simulink model "TCS_Simulation"  (R2023b)
settings: Solver=FixedStepAuto  StartTime=0.0  StopTime=5  FixedStep=0.03  RelTol=1e-3
undefined symbols (not defined in the file): Ion, Lithium, sigbuilder_block
libraries: spsMosfetLib x24, fl_lib x20, nesl_utility x19, sdl_lib x12, slpidlib x5, spsBatteryLib x4, spsSeriesRLCBranchLib x4, spsPermanentMagnetSynchronousMachineLib x4, spspowerguiLib x1
(part 1 of 3)
settings Model: Creator=hp  LastModifiedBy=ADMIN
settings DebuggingCC: UnconnectedInputMsg=warning  UnconnectedOutputMsg=warning  UnconnectedLineMsg=warning
settings ModelReferenceCC: EnableRefExpFcnMdlSchedulingChecks=on
settings RTWCC: DLArmComputeVersion=19.05

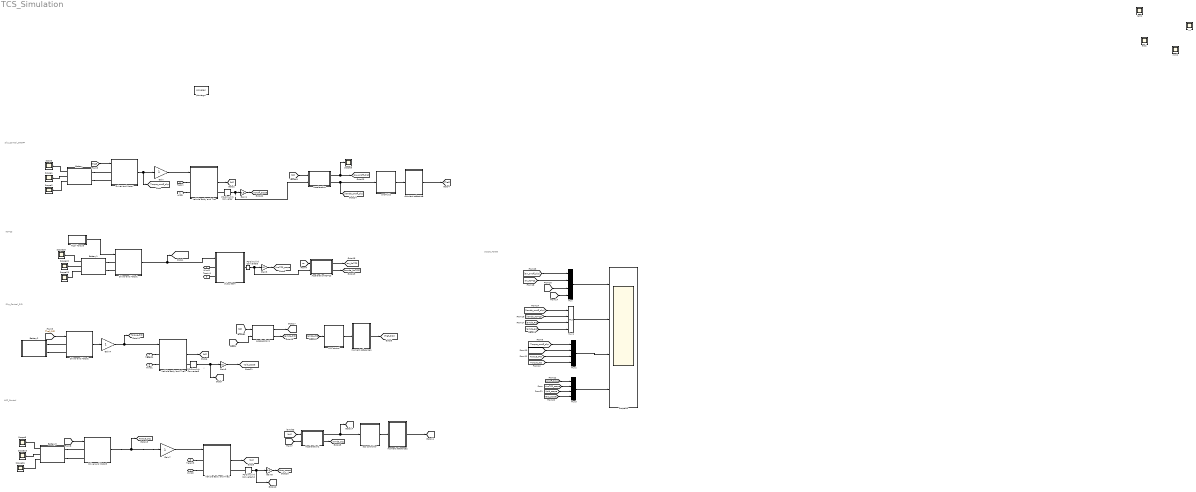
== system TCS_Simulation ==
  note: Scope_4Data
  note: Slip_Control_ONOFF
  note: NoTCS
  note: Slip_Control_PID
  note: ACC_Control
  note: v
  note: v
  Acceleration : Subsystem
  Acceleration1 : Subsystem
  Acceleration2 : Subsystem
  AccelerationNOTCS : Subsystem
  Battery : Subsystem
  Battery1 : Subsystem
  Battery2 : Subsystem
  Battery3 : Subsystem
  Driver and Motor : Subsystem
  Driver and Motor1 : Subsystem
  Driver and Motor2 : Subsystem
  Driver and Motor3 : Subsystem
  Gain : Gain
  Gain{1,3,5,8} (4 alike) : Gain  Gain=3.6
  Gain4 : Gain
  Gain7 : Gain
  High Torque : Subsystem  Tag=STV Subsys  LoadFcn=sigbuilder_block('load');  StartFcn=sigbuilder_block('start');  StopFcn=sigbuilder_block('stop');  ClipboardFcn=sigbuilder_block('clipboard');  mask(Sigbuilder block){tuvar=[0:10]}
      mask help: Simulink:masks:SigbuilderBlock_MD
      mask init:
      | if ~strcmp(get_param(bdroot(gcbh),'SimulationStatus'),'stopped') tuvar = sigbuilder_block('maskInit'); end
      settings: CopyFcn=sigbuilder_block('copy');  DeleteFcn=sigbuilder_block('delete');  ModelCloseFcn=sigbuilder_block('modelClose');  PreSaveFcn=sigbuilder_block('preSave');  PauseFcn=sigbuilder_block('pause');  ContinueFcn=sigbuilder_block('continue');  NameChangeFcn=sigbuilder_block('namechange');  OpenFcn=sigbuilder_block('open',[5.4 36 1141.2 516.6 ]);  CloseFcn=sigbuilder_block('close');
      mask Display: plot(0, 0, 100, 100,[2, 2, 32, 32, 2], [68, 8, 8, 68, 68],[32, 2], [38, 38], [32, 19, 2],[53, 60, 44], [32, 17, 17, 2],[16, 16, 31, 31]);txt = getActiveGroup(gcbh);text(2, 100, txt,'verticalAlignment', 'top');
  Mux{,1..3} (4 alike) : Mux
  PID control : Subsystem
  PS-Simulink Converter : nesl_utility/PS-Simulink Converter  PhysicalDomain=network_engine_domain  SubClassName=ps_output  LeftPortType=input  RightPortType=output  PseudoPeriodic=off  Frequencies=[]  VectorFormat=1-D array  Unit=1  AffineConversion=off
  PS-Simulink Converter12 : nesl_utility/PS-Simulink Converter  PhysicalDomain=network_engine_domain  SubClassName=ps_output  LeftPortType=input  RightPortType=output  PseudoPeriodic=off  Frequencies=[]  VectorFormat=1-D array  Unit=1  AffineConversion=off
  PS-Simulink Converter3 : nesl_utility/PS-Simulink Converter  PhysicalDomain=network_engine_domain  SubClassName=ps_output  LeftPortType=input  RightPortType=output  PseudoPeriodic=off  Frequencies=[]  VectorFormat=1-D array  Unit=inherit  AffineConversion=off
  PS-Simulink Converter8 : nesl_utility/PS-Simulink Converter  PhysicalDomain=network_engine_domain  SubClassName=ps_output  LeftPortType=input  RightPortType=output  PseudoPeriodic=off  Frequencies=[]  VectorFormat=1-D array  Unit=1  AffineConversion=off
  Scope{,1..3,8,16,18,22..23,26} (10 alike) : Scope
  Scope36 : Scope  NumInputPorts=4
  Subsystem : Subsystem
  Vehicle Body and Tire : Subsystem
  Vehicle Body and Tire1 : Subsystem
  Vehicle Body and Tire2 : Subsystem
  acc controller : Subsystem
  acc1 : Scope  NumInputPorts=4
  lam1 : Scope  NumInputPorts=4
  mm2 : Scope  NumInputPorts=4
  moment reference : Subsystem
  moment reference1 : Subsystem
  moment reference2 : Subsystem
  onoff slip : Subsystem
  powergui : spspowerguiLib/powergui  Priority=1  SimulationMode=Discrete  SampleTime=0.03  frequency=60  Iterations=50  frequencyindice=0  Pbase=100e6  ErrMax=1e-4  UnitsV=kV  UnitsW=MW  buscounter=0  FunctionMessages=off  echomessages=off  EnableUseOfTLC=off  CurrentSourceSwitches=off  DisableSnubberDevices=off  DisableRonSwitches=off  DisableVfSwitches=off  DisplayEquations=off  AutomaticDiscreteSolvers=off  SolverType=Tustin/Backward Euler (TBE)  Interpol=off  ExternalGateDelay=off  methode=off  Ts=10  x0status=blocks  SPID=off  SwTol=0  HookPort=off  NonlinearTolerance=1e-4  nMaxIteration=100  ContinueOnMaxIteration=off  RestoreLinks=warning  ResistiveCurrentMeasurement=off  Frange=[0:2:500]  Ylog=off  Xlog=on  ShowGrid=off  save=off  variable=ZData  structure=0  ZoomFFT=off  StartTime=0.0  cycles=1  DisplayStyle=1  fundamental=60  FreqAxis=off  MaxFrequency=1000  frequencyindicesteady=1  RmsSteady=1  display=off
  vv : Scope  NumInputPorts=4
  " Wind" : PMIOPort  Side=Left
  Terain : PMIOPort  Port=2  Side=Right
  Terain1 : PMIOPort  Port=3  Side=Left
  Wind1 : PMIOPort  Port=4  Side=Left
  " Wind1" : PMIOPort  Port=5  Side=Left
  Terain2 : PMIOPort  Port=6  Side=Right
  " Wind2" : PMIOPort  Port=7  Side=Left
  Terain3 : PMIOPort  Port=8  Side=Right
  tag scope: Torque_PID=global, Torque_acc=global, Torque_onoff_slip=global, VnoTCS_scope=global, Vonoff_Scope=global, Vpid_scope=global, aw_NoTCS=global, aw_PID=global, aw_acc=global, lamda_acc=global
  wires:
  moment reference/1(Tref) -> [Tref]
  Driver and Motor1/1(Torque) -> [Torque_NoTCS], Subsystem/1(Torque)
  Battery1/2(current) -> Scope22/1
  Battery1/3(Voltage) -> Scope23/1
  Battery/2(current) -> Scope1/1
  Battery1/1(SOC) -> Scope18/1
  [ss] -> AccelerationNOTCS/1(lamda1)
  [s1] -> Acceleration/1(lamda1)
  PS-Simulink Converter3/1 -> AccelerationNOTCS/2(Vx), Gain3/1
  Battery/1(SOC) -> Scope/1
  Gain/1 -> Vehicle Body and Tire/1(Torque)
  [Tref] -> Driver and Motor/1(Tref)
  PS-Simulink Converter/1 -> Acceleration/2(Vx), Gain1/1
  Driver and Motor/1(Torque) -> [Torque_onoff_slip], Gain/1
  Gain1/1 -> [Vonoff_Scope]
  Battery/3(Voltage) -> Scope2/1
  onoff slip/1(s) -> moment reference/1(S)
  Acceleration/2(lamda) -> [lamda_onoff_slip], onoff slip/1(lamda)
  AccelerationNOTCS/1(aw) -> [aw_NoTCS]
  AccelerationNOTCS/2(lamdaNoTCS) -> [lamda_NoTCS]
  Acceleration/1(aw) -> Scope3/1, [aw_onoff_slip]
  High Torque/1(Signal 1) -> Driver and Motor1/1(Tref)
  Vehicle Body and Tire/2(S) -> [s1]
  Vehicle Body and Tire1/2(s) -> [s2]
  Gain5/1 -> [Vpid_scope]
  PS-Simulink Converter8/1 -> [Vxpid], Gain5/1
  moment reference1/1(Tref) -> [Tref_PID]
  [Vxpid] -> Acceleration1/2(Vx)
  [Tref_PID] -> Driver and Motor2/1(Tref)
  Gain4/1 -> [Torque_PID], Vehicle Body and Tire1/1(Torque)
  Driver and Motor2/1(Torque) -> Gain4/1
  Acceleration1/2(lamda) -> [lamda_PID]
  PID control/1(s) -> moment reference1/1(S)
  [s2] -> Acceleration1/1(lamda1)
  Acceleration1/1(aw) -> [aw_PID]
  moment reference2/1(Tref) -> [Trefacc]
  [Vxacc] -> Acceleration2/2(Vx)
  Acceleration2/1(aw) -> acc controller/1(aw), [aw_acc]
  Battery3/3(Voltage) -> Scope26/1
  Vehicle Body and Tire2/2(s4) -> [s4]
  Acceleration2/2(lamda) -> [lamda_acc]
  PS-Simulink Converter12/1 -> Gain8/1, [Vxacc]
  Gain7/1 -> Vehicle Body and Tire2/1(Torque)
  acc controller/1(s) -> moment reference2/1(S)
  [s4] -> Acceleration2/1(lamda1)
  Battery3/2(current) -> Scope16/1
  Gain8/1 -> [Vacc_scope]
  [Trefacc] -> Driver and Motor3/1(Tref)
  Battery3/1(SOC) -> Scope8/1
  Driver and Motor3/1(Torque) -> Gain7/1, [Torque_acc]
  Mux/1 -> Scope36/1
  Mux1/1 -> Scope36/2
  Mux2/1 -> Scope36/3
  Mux3/1 -> Scope36/4
  [VnoTCS_scope] -> Mux3/2
  [Torque_onoff_slip] -> Mux2/1
  Gain3/1 -> [VnoTCS_scope]
  [Torque_NoTCS] -> Mux2/2
  [Torque_PID] -> Mux2/3
  [Torque_acc] -> Mux2/4
  [lamda_acc] -> Mux1/4
  [aw_acc] -> Mux/4
  [aw_PID] -> Mux/3
  [lamda_PID] -> PID control/1(lamda)
  [lamda_PID] -> Mux1/3
  [aw_NoTCS] -> Mux/2
  [lamda_NoTCS] -> Mux1/2
  [Vacc_scope] -> Mux3/4
  [Vpid_scope] -> Mux3/3
  [Vonoff_Scope] -> Mux3/1
  [aw_onoff_slip] -> Mux/1
  [lamda_onoff_slip] -> Mux1/1
  connections:
  Battery/LConn2 -- Driver and Motor/LConn2
  Battery/LConn1 -- Driver and Motor/LConn1
  " Wind"/RConn1 -- Vehicle Body and Tire/LConn2
  Terain/RConn1 -- Vehicle Body and Tire/LConn1
  PS-Simulink Converter/LConn1 -- Vehicle Body and Tire/RConn1
  Battery1/LConn1 -- Driver and Motor1/LConn1
  Battery1/LConn2 -- Driver and Motor1/LConn2
  Battery2/LConn2 -- Driver and Motor2/LConn2
  " Wind1"/RConn1 -- Vehicle Body and Tire1/LConn2
  Terain2/RConn1 -- Vehicle Body and Tire1/LConn1
  PS-Simulink Converter8/LConn1 -- Vehicle Body and Tire1/RConn1
  Battery2/LConn1 -- Driver and Motor2/LConn1
  Battery3/LConn1 -- Driver and Motor3/LConn1
  PS-Simulink Converter12/LConn1 -- Vehicle Body and Tire2/RConn1
  Battery3/LConn2 -- Driver and Motor3/LConn2
  " Wind2"/RConn1 -- Vehicle Body and Tire2/LConn2
  Terain3/RConn1 -- Vehicle Body and Tire2/LConn1
  Subsystem/RConn1 -- PS-Simulink Converter3/LConn1
  Subsystem/LConn1 -- Wind1/RConn1
  Subsystem/LConn2 -- Terain1/RConn1

== system TCS_Simulation/Acceleration ==
  note: W
  lamda1 : Inport
  Vx : Inport  Port=2
  Add : Sum
  Add1 : Sum  Inputs=+-
  Constant : Constant
  Derivative1 : Derivative
  Divide : Product  Inputs=*/
  Gain : Gain  Gain=1/0.22
  Product : Product
  Saturation : Saturate  UpperLimit=1  LowerLimit=0
  Scope1 : Scope
  Scope2 : Scope
  r : Gain  Gain=0.22
  wheel speed1 : Scope
  aw : Outport
  lamda : Outport  Port=2
  wires:
  Gain/1 -> r/1, wheel speed1/1
  lamda1/1 -> Product/1
  Product/1 -> Add/1
  r/1 -> Derivative1/1
  Constant/1 -> Add1/1
  Divide/1 -> Add1/2
  Add/1 -> Divide/2, Scope2/1, Gain/1
  Add1/1 -> Scope1/1, Saturation/1
  Vx/1 -> Divide/1, Add/2, Product/2
  Saturation/1 -> lamda/1
  Derivative1/1 -> aw/1

== system TCS_Simulation/Acceleration1 ==
  note: W
  lamda1 : Inport
  Vx : Inport  Port=2
  Add : Sum
  Add1 : Sum  Inputs=+-
  Constant : Constant
  Derivative1 : Derivative
  Divide : Product  Inputs=*/
  Gain : Gain  Gain=1/0.22
  Product : Product
  Saturation : Saturate  UpperLimit=1  LowerLimit=0
  Scope1 : Scope
  Scope2 : Scope
  r : Gain  Gain=0.22
  wheel speed1 : Scope
  aw : Outport
  lamda : Outport  Port=2
  wires:
  Gain/1 -> r/1, wheel speed1/1
  lamda1/1 -> Product/1
  Product/1 -> Add/1
  r/1 -> Derivative1/1
  Constant/1 -> Add1/1
  Divide/1 -> Add1/2
  Add/1 -> Divide/2, Scope2/1, Gain/1
  Add1/1 -> Scope1/1, Saturation/1
  Vx/1 -> Divide/1, Add/2, Product/2
  Saturation/1 -> lamda/1
  Derivative1/1 -> aw/1

== system TCS_Simulation/Acceleration2 ==
  note: W
  lamda1 : Inport
  Vx : Inport  Port=2
  Add : Sum
  Add1 : Sum  Inputs=+-
  Constant : Constant
  Derivative1 : Derivative
  Divide : Product  Inputs=*/
  Gain : Gain  Gain=1/0.22
  Product : Product
  Saturation : Saturate  UpperLimit=1  LowerLimit=0
  Scope1 : Scope
  Scope2 : Scope
  r : Gain  Gain=0.22
  wheel speed1 : Scope
  aw : Outport
  lamda : Outport  Port=2
  wires:
  Gain/1 -> r/1, wheel speed1/1
  lamda1/1 -> Product/1
  Product/1 -> Add/1
  r/1 -> Derivative1/1
  Constant/1 -> Add1/1
  Divide/1 -> Add1/2
  Add/1 -> Divide/2, Scope2/1, Gain/1
  Add1/1 -> Scope1/1, Saturation/1
  Vx/1 -> Divide/1, Add/2, Product/2
  Saturation/1 -> lamda/1
  Derivative1/1 -> aw/1

== system TCS_Simulation/AccelerationNOTCS ==
  note: Wr
  lamda1 : Inport
  Vx : Inport  Port=2
  Add : Sum
  Add1 : Sum  Inputs=+-
  Constant : Constant
  Derivative : Derivative
  Divide : Product  Inputs=*/
  Product : Product
  Scope1 : Scope
  Scope2 : Scope
  aw : Outport
  lamdaNoTCS : Outport  Port=2
  wires:
  Derivative/1 -> aw/1
  lamda1/1 -> Product/1
  Product/1 -> Add/1
  Add/1 -> Derivative/1, Divide/2, Scope2/1
  Constant/1 -> Add1/1
  Divide/1 -> Add1/2
  Add1/1 -> lamdaNoTCS/1
  Vx/1 -> Scope1/1, Divide/1, Product/2, Add/2

== system TCS_Simulation/Battery ==
  Battery : spsBatteryLib/Battery  BatType=Lithium-Ion  ShowTempParam=off  ThermalPreset=no  ShowAgeParam=off  NomV=50.4  NomQ=22  SOC=100  Batt_Tr=30  PresetModel=on  MaxQ=22  MinV=37.8  FullV=58.665  Dis_rate=9.5652  R=0.022909  Normal_OP=19.8957  expZone="[54.4514      1.08087]"  current=[6.5 13 32.5]  Units=Time  Tci=20  NomT=25  T2=0  MaxQ2=2.208  FullV2=3.45  Normal_OP2=2.8  expZone2="[3.22        0.23]"  Rca=0.6  ti=1000  Dp=0  Neq0=0  Tsim=1e6  Ta1=25  Qeol=5.4*0.9  Reol=0.013333*1.2  Char_age=[2.3478, 3]  Dis_age=[2.3478, 10]  N1=1500  N2=10500  N3=1000  N4=1400  Ta2=45  N5=950
  Bus Selector : BusSelector  OutputSignals=SOC (%),Current (A),Voltage (V)
  Series RLC Branch : spsSeriesRLCBranchLib/Series RLC Branch  LConnTagsString=__new0  RConnTagsString=__new0  BranchType=C  Resistance=1  Inductance=1e-3  SetiL0=off  InitialCurrent=0  Capacitance=75e-3  Setx0=off  InitialVoltage=0  Measurements=None
  " Positive" : PMIOPort  Side=Left
  Negative : PMIOPort  Port=2  Side=Left
  SOC : Outport
  current : Outport  Port=2
  Voltage : Outport  Port=3
  wires:
  Battery/1 -> Bus Selector/1
  Bus Selector/1 -> SOC/1  "<SOC (%)>"
  Bus Selector/2 -> current/1  "<Current (A)>"
  Bus Selector/3 -> Voltage/1  "<Voltage (V)>"
  connections:
  " Positive"/RConn1 -- Battery/LConn1 -- Series RLC Branch/LConn1
  Negative/RConn1 -- Series RLC Branch/RConn1 -- Battery/LConn2

== system TCS_Simulation/Battery1 ==
  Battery : spsBatteryLib/Battery  BatType=Lithium-Ion  ShowTempParam=off  ThermalPreset=no  ShowAgeParam=off  NomV=50.4  NomQ=22  SOC=100  Batt_Tr=30  PresetModel=on  MaxQ=22  MinV=37.8  FullV=58.665  Dis_rate=9.5652  R=0.022909  Normal_OP=19.8957  expZone="[54.4514      1.08087]"  current=[6.5 13 32.5]  Units=Time  Tci=20  NomT=25  T2=0  MaxQ2=2.208  FullV2=3.45  Normal_OP2=2.8  expZone2="[3.22        0.23]"  Rca=0.6  ti=1000  Dp=0  Neq0=0  Tsim=1e6  Ta1=25  Qeol=5.4*0.9  Reol=0.013333*1.2  Char_age=[2.3478, 3]  Dis_age=[2.3478, 10]  N1=1500  N2=10500  N3=1000  N4=1400  Ta2=45  N5=950
  Bus Selector : BusSelector  OutputSignals=SOC (%),Current (A),Voltage (V)
  Series RLC Branch : spsSeriesRLCBranchLib/Series RLC Branch  LConnTagsString=__new0  RConnTagsString=__new0  BranchType=C  Resistance=1  Inductance=1e-3  SetiL0=off  InitialCurrent=0  Capacitance=75e-3  Setx0=off  InitialVoltage=0  Measurements=None
  " Positive" : PMIOPort  Side=Left
  Negative : PMIOPort  Port=2  Side=Left
  SOC : Outport
  current : Outport  Port=2
  Voltage : Outport  Port=3
  wires:
  Battery/1 -> Bus Selector/1
  Bus Selector/1 -> SOC/1  "<SOC (%)>"
  Bus Selector/2 -> current/1  "<Current (A)>"
  Bus Selector/3 -> Voltage/1  "<Voltage (V)>"
  connections:
  " Positive"/RConn1 -- Battery/LConn1 -- Series RLC Branch/LConn1
  Negative/RConn1 -- Series RLC Branch/RConn1 -- Battery/LConn2

== system TCS_Simulation/Battery2 ==
  Battery : spsBatteryLib/Battery  BatType=Lithium-Ion  ShowTempParam=off  ThermalPreset=no  ShowAgeParam=off  NomV=50.4  NomQ=22  SOC=100  Batt_Tr=30  PresetModel=on  MaxQ=22  MinV=37.8  FullV=58.665  Dis_rate=9.5652  R=0.022909  Normal_OP=19.8957  expZone="[54.4514      1.08087]"  current=[6.5 13 32.5]  Units=Time  Tci=20  NomT=25  T2=0  MaxQ2=2.208  FullV2=3.45  Normal_OP2=2.8  expZone2="[3.22        0.23]"  Rca=0.6  ti=1000  Dp=0  Neq0=0  Tsim=1e6  Ta1=25  Qeol=5.4*0.9  Reol=0.013333*1.2  Char_age=[2.3478, 3]  Dis_age=[2.3478, 10]  N1=1500  N2=10500  N3=1000  N4=1400  Ta2=45  N5=950
  Bus Selector : BusSelector  OutputSignals=SOC (%),Current (A),Voltage (V)
  Series RLC Branch : spsSeriesRLCBranchLib/Series RLC Branch  LConnTagsString=__new0  RConnTagsString=__new0  BranchType=C  Resistance=1  Inductance=1e-3  SetiL0=off  InitialCurrent=0  Capacitance=75e-3  Setx0=off  InitialVoltage=0  Measurements=None
  " Positive" : PMIOPort  Side=Left
  Negative : PMIOPort  Port=2  Side=Left
  SOC : Outport
  current : Outport  Port=2
  Voltage : Outport  Port=3
  wires:
  Battery/1 -> Bus Selector/1
  Bus Selector/1 -> SOC/1  "<SOC (%)>"
  Bus Selector/2 -> current/1  "<Current (A)>"
  Bus Selector/3 -> Voltage/1  "<Voltage (V)>"
  connections:
  " Positive"/RConn1 -- Battery/LConn1 -- Series RLC Branch/LConn1
  Negative/RConn1 -- Series RLC Branch/RConn1 -- Battery/LConn2

== system TCS_Simulation/Battery3 ==
  Battery : spsBatteryLib/Battery  BatType=Lithium-Ion  ShowTempParam=off  ThermalPreset=no  ShowAgeParam=off  NomV=50.4  NomQ=22  SOC=100  Batt_Tr=30  PresetModel=on  MaxQ=22  MinV=37.8  FullV=58.665  Dis_rate=9.5652  R=0.022909  Normal_OP=19.8957  expZone="[54.4514      1.08087]"  current=[6.5 13 32.5]  Units=Time  Tci=20  NomT=25  T2=0  MaxQ2=2.208  FullV2=3.45  Normal_OP2=2.8  expZone2="[3.22        0.23]"  Rca=0.6  ti=1000  Dp=0  Neq0=0  Tsim=1e6  Ta1=25  Qeol=5.4*0.9  Reol=0.013333*1.2  Char_age=[2.3478, 3]  Dis_age=[2.3478, 10]  N1=1500  N2=10500  N3=1000  N4=1400  Ta2=45  N5=950
  Bus Selector : BusSelector  OutputSignals=SOC (%),Current (A),Voltage (V)
  Series RLC Branch : spsSeriesRLCBranchLib/Series RLC Branch  LConnTagsString=__new0  RConnTagsString=__new0  BranchType=C  Resistance=1  Inductance=1e-3  SetiL0=off  InitialCurrent=0  Capacitance=75e-3  Setx0=off  InitialVoltage=0  Measurements=None
  " Positive" : PMIOPort  Side=Left
  Negative : PMIOPort  Port=2  Side=Left
  SOC : Outport
  current : Outport  Port=2
  Voltage : Outport  Port=3
  wires:
  Battery/1 -> Bus Selector/1
  Bus Selector/1 -> SOC/1  "<SOC (%)>"
  Bus Selector/2 -> current/1  "<Current (A)>"
  Bus Selector/3 -> Voltage/1  "<Voltage (V)>"
  connections:
  " Positive"/RConn1 -- Battery/LConn1 -- Series RLC Branch/LConn1
  Negative/RConn1 -- Series RLC Branch/RConn1 -- Battery/LConn2

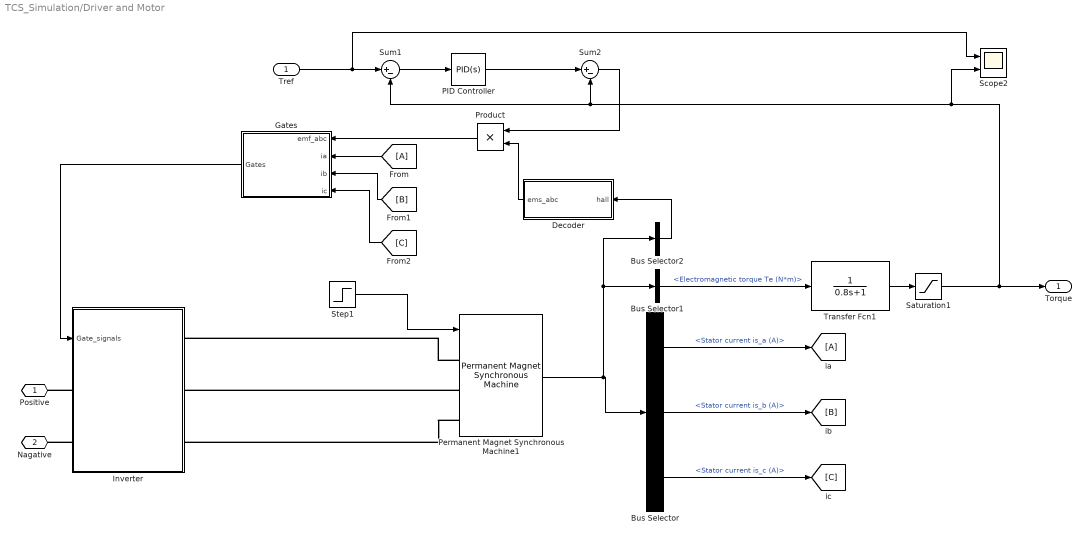
== system TCS_Simulation/Driver and Motor ==
  Tref : Inport
  Bus Selector : BusSelector  OutputSignals=Stator current is_a (A),Stator current is_b (A),Stator current is_c (A)
  Bus Selector1 : BusSelector  OutputSignals=Electromagnetic torque Te (N*m)
  Bus Selector2 : BusSelector  OutputSignals=Hall effect signal h_a,Hall effect signal h_b,Hall effect signal h_c  OutputAsBus=on
  Decoder : Subsystem
  From : From
  Gates : Subsystem
  Inverter : Subsystem
  PID Controller : slpidlib/PID Controller  Controller=PID  Form=Parallel  TimeDomain=Continuous-time  UseExternalTs=off  SampleTime=-1  IntegratorMethod=Forward Euler  FilterMethod=Forward Euler  ControllerParametersSource=internal  P=100  I=10  UseKiTs=off  D=1  N=100  UseFilter=on  TunerSelectOption=Transfer Function Based (PID Tuner App)  InitialConditionSource=internal  InitialConditionForIntegrator=0  InitialConditionForFilter=0  DifferentiatorICPrevScaledInput=0  ExternalReset=none  TrackingMode=off  Kt=1  LimitOutput=off  SatLimitsSource=internal  UpperSaturationLimit=inf  LowerSaturationLimit=-inf  LinearizeAsGain=on  AntiWindupMode=none  Kb=1  LimitIntegrator=off  UpperIntegratorSaturationLimit=inf  LowerIntegratorSaturationLimit=-inf  POutMin=[]  POutMax=[]  IOutMin=[]  IOutMax=[]  DOutMin=[]  DOutMax=[]  NOutMin=[]  NOutMax=[]  SumOutMin=[]  SumOutMax=[]  SaturationOutMin=[]  SaturationOutMax=[]  PParamMin=[]  PParamMax=[]  IParamMin=[]  IParamMax=[]  DParamMin=[]  DParamMax=[]  NParamMin=[]  NParamMax=[]  KbParamMin=[]  KbParamMax=[]  KtParamMin=[]  KtParamMax=[]  KbOutMin=[]  KbOutMax=[]  KtOutMin=[]  KtOutMax=[]  IntegratorOutMin=[]  IntegratorOutMax=[]  FilterOutMin=[]  FilterOutMax=[]  SumI1OutMin=[]  SumI1OutMax=[]  SumI2OutMin=[]  SumI2OutMax=[]  SumI3OutMin=[]  SumI3OutMax=[]  SumI4OutMin=[]  SumI4OutMax=[]  SumDOutMin=[]  SumDOutMax=[]  DifferentiatorOutMin=[]  DifferentiatorOutMax=[]  FilterDiffOutCoefMin=[]  FilterDiffOutCoefMax=[]  ReciprocalOutMin=[]  ReciprocalOutMax=[]  SumDenOutMin=[]  SumDenOutMax=[]  SumNumOutMin=[]  SumNumOutMax=[]  DivideOutMin=[]  DivideOutMax=[]  UdiffTsProdOutMin=[]  UdiffTsProdOutMax=[]  NTsProdOutMin=[]  NTsProdOutMax=[]  UintegralTsProdOutMin=[]  UintegralTsProdOutMax=[]  UngainTsProdOutMin=[]  UngainTsProdOutMax=[]  ClampingZeroOutDataTypeStr=Inherit: Inherit via back propagation  ClampingZeroOutMin=[]  ClampingZeroOutMax=[]  FilterDenConstantOutDataTypeStr=Inherit: Inherit via back propagation  FilterDenConstantOutMin=[]  FilterDenConstantOutMax=[]  PCopyOutDataTypeStr=Inherit: Inherit via back propagation  PCopyOutMin=[]  PCopyOutMax=[]  NCopyOutDataTypeStr=Inherit: Inherit via back propagation  NCopyOutMin=[]  NCopyOutMax=[]  IntegratorContinuousStateAttributes=''  IntegratorStateMustResolveToSignalObject=off  IntegratorRTWStateStorageClass=Auto  FilterContinuousStateAttributes=''  FilterStateMustResolveToSignalObject=off  FilterRTWStateStorageClass=Auto  ParallelPVariant=InternalParameters  IdealPVariant=Disabled  IVariant=InternalParameters  DVariant=InternalParameters  IntegratorVariant=Continuous  SatVariant=Disabled  AWVariant=Passthrough  PCopyVariant=Disabled  TRVariant=Disabled  FdbkBlocksVariant=Forward  IdealPFdbkVariant=Disabled  SatFdbkVariant=Disabled  DerivativeFilterVariant=ContFilter  NVariant=InternalParameters  NCopyVariant=Disabled  FilterICVariant=InternalICsFilter  IntegratorICVariant=InternalICs  ExternalResetVariant=Disabled  TRSumVariant=Passthrough  SumFdbkVariant=Disabled  SumVariant=Sum_PID  TsampFilterVariant=InternalTs  TsampNgainVariant=Passthrough  TsampIntegralVariant=Disabled_SignalSpec  ExternalSaturationOutDataTypeStr=Inherit: Same as second input
  Permanent Magnet Synchronous Machine1 : spsPermanentMagnetSynchronousMachineLib/Permanent Magnet Synchronous Machine  NbPhases=3  FluxDistribution=Trapezoidal  RotorType=Round  MechanicalLoad=Speed w  PresetModel=No  ShowDetailedParameters=on  MeasurementBus=off  Resistance=0.0485  Inductance=8.5e-3  dqInductances=[8.5e-3,8.5e-3]  La=0.000395  MachineConstant=Flux linkage established by magnets (V.s)  Flux=0.1194  VoltageCst=150.0425  TorqueCst=1.4328  Flat=120  Mechanical=[0.0027 0.0004924 4 0]  PolePairs=6  InitialConditions=[0,0, 0,0]  InitialConditions5ph=[0 0 0 0 0 0]  RefAngle=90 degrees behind phase A axis (modified Park)  IterativeDiscreteModel=Trapezoidal non iterative  TsBlock=-1  TsPowergui=0
  Product : Product
  Saturation1 : Saturate  UpperLimit=10000  LowerLimit=0
  Scope2 : Scope  NumInputPorts=2
  Step1 : Step  Time=100  After=200  SampleTime=0
  Sum1 : Sum  Inputs=|+-
  Sum2 : Sum  Inputs=|+-
  Transfer Fcn1 : TransferFcn  Denominator=[0.8 1]
  ia : Goto
  Positive : PMIOPort  Side=Left
  Nagative : PMIOPort  Port=2  Side=Left
  Torque : Outport
  wires:
  Bus Selector/3 -> [C]  "<Stator current is_c (A)>"
  Bus Selector2/1 -> Decoder/1(hall)
  [B] -> Gates/3(ib)
  Gates/1(Gates) -> Inverter/1(Gate_signals)
  Permanent Magnet Synchronous Machine1/1 -> Bus Selector1/1, Bus Selector2/1, Bus Selector/1
  Bus Selector/1 -> ia/1  "<Stator current is_a (A)>"
  Bus Selector/2 -> [B]  "<Stator current is_b (A)>"
  [C] -> Gates/4(ic)
  From/1 -> Gates/2(ia)
  Bus Selector1/1 -> Transfer Fcn1/1  "<Electromagnetic torque Te (N*m)>"
  Step1/1 -> Permanent Magnet Synchronous Machine1/1
  Decoder/1(ems_abc) -> Product/2
  Product/1 -> Gates/1(emf_abc)
  Sum1/1 -> PID Controller/1
  Tref/1 -> Scope2/1, Sum1/1
  PID Controller/1 -> Sum2/1
  Sum2/1 -> Product/1
  Transfer Fcn1/1 -> Saturation1/1
  Saturation1/1 -> Torque/1, Sum1/2, Sum2/2, Scope2/2
  connections:
  Inverter/LConn1 -- Positive/RConn1
  Inverter/LConn2 -- Nagative/RConn1
  Permanent Magnet Synchronous Machine1/LConn1 -- Inverter/RConn1
  Permanent Magnet Synchronous Machine1/LConn2 -- Inverter/RConn2
  Permanent Magnet Synchronous Machine1/LConn3 -- Inverter/RConn3

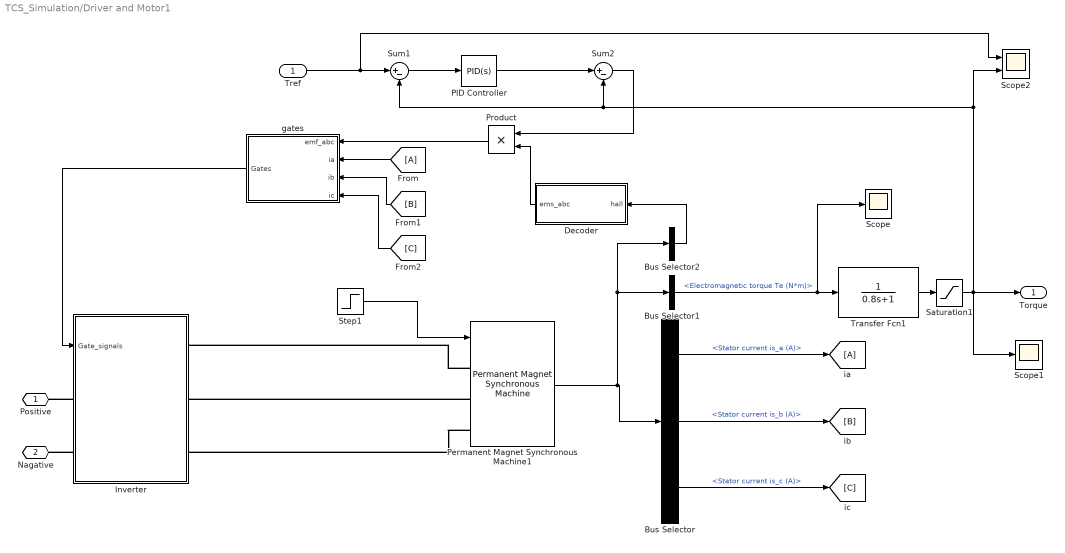
== system TCS_Simulation/Driver and Motor1 ==
  Tref : Inport
  Bus Selector : BusSelector  OutputSignals=Stator current is_a (A),Stator current is_b (A),Stator current is_c (A)
  Bus Selector1 : BusSelector  OutputSignals=Electromagnetic torque Te (N*m)
  Bus Selector2 : BusSelector  OutputSignals=Hall effect signal h_a,Hall effect signal h_b,Hall effect signal h_c  OutputAsBus=on
  Decoder : Subsystem
  From : From
  Inverter : Subsystem
  PID Controller : slpidlib/PID Controller  Controller=PID  Form=Parallel  TimeDomain=Continuous-time  UseExternalTs=off  SampleTime=-1  IntegratorMethod=Forward Euler  FilterMethod=Forward Euler  ControllerParametersSource=internal  P=100  I=10  UseKiTs=off  D=1  N=100  UseFilter=on  TunerSelectOption=Transfer Function Based (PID Tuner App)  InitialConditionSource=internal  InitialConditionForIntegrator=0  InitialConditionForFilter=0  DifferentiatorICPrevScaledInput=0  ExternalReset=none  TrackingMode=off  Kt=1  LimitOutput=off  SatLimitsSource=internal  UpperSaturationLimit=inf  LowerSaturationLimit=-inf  LinearizeAsGain=on  AntiWindupMode=none  Kb=1  LimitIntegrator=off  UpperIntegratorSaturationLimit=inf  LowerIntegratorSaturationLimit=-inf  POutMin=[]  POutMax=[]  IOutMin=[]  IOutMax=[]  DOutMin=[]  DOutMax=[]  NOutMin=[]  NOutMax=[]  SumOutMin=[]  SumOutMax=[]  SaturationOutMin=[]  SaturationOutMax=[]  PParamMin=[]  PParamMax=[]  IParamMin=[]  IParamMax=[]  DParamMin=[]  DParamMax=[]  NParamMin=[]  NParamMax=[]  KbParamMin=[]  KbParamMax=[]  KtParamMin=[]  KtParamMax=[]  KbOutMin=[]  KbOutMax=[]  KtOutMin=[]  KtOutMax=[]  IntegratorOutMin=[]  IntegratorOutMax=[]  FilterOutMin=[]  FilterOutMax=[]  SumI1OutMin=[]  SumI1OutMax=[]  SumI2OutMin=[]  SumI2OutMax=[]  SumI3OutMin=[]  SumI3OutMax=[]  SumI4OutMin=[]  SumI4OutMax=[]  SumDOutMin=[]  SumDOutMax=[]  DifferentiatorOutMin=[]  DifferentiatorOutMax=[]  FilterDiffOutCoefMin=[]  FilterDiffOutCoefMax=[]  ReciprocalOutMin=[]  ReciprocalOutMax=[]  SumDenOutMin=[]  SumDenOutMax=[]  SumNumOutMin=[]  SumNumOutMax=[]  DivideOutMin=[]  DivideOutMax=[]  UdiffTsProdOutMin=[]  UdiffTsProdOutMax=[]  NTsProdOutMin=[]  NTsProdOutMax=[]  UintegralTsProdOutMin=[]  UintegralTsProdOutMax=[]  UngainTsProdOutMin=[]  UngainTsProdOutMax=[]  ClampingZeroOutDataTypeStr=Inherit: Inherit via back propagation  ClampingZeroOutMin=[]  ClampingZeroOutMax=[]  FilterDenConstantOutDataTypeStr=Inherit: Inherit via back propagation  FilterDenConstantOutMin=[]  FilterDenConstantOutMax=[]  PCopyOutDataTypeStr=Inherit: Inherit via back propagation  PCopyOutMin=[]  PCopyOutMax=[]  NCopyOutDataTypeStr=Inherit: Inherit via back propagation  NCopyOutMin=[]  NCopyOutMax=[]  IntegratorContinuousStateAttributes=''  IntegratorStateMustResolveToSignalObject=off  IntegratorRTWStateStorageClass=Auto  FilterContinuousStateAttributes=''  FilterStateMustResolveToSignalObject=off  FilterRTWStateStorageClass=Auto  ParallelPVariant=InternalParameters  IdealPVariant=Disabled  IVariant=InternalParameters  DVariant=InternalParameters  IntegratorVariant=Continuous  SatVariant=Disabled  AWVariant=Passthrough  PCopyVariant=Disabled  TRVariant=Disabled  FdbkBlocksVariant=Forward  IdealPFdbkVariant=Disabled  SatFdbkVariant=Disabled  DerivativeFilterVariant=ContFilter  NVariant=InternalParameters  NCopyVariant=Disabled  FilterICVariant=InternalICsFilter  IntegratorICVariant=InternalICs  ExternalResetVariant=Disabled  TRSumVariant=Passthrough  SumFdbkVariant=Disabled  SumVariant=Sum_PID  TsampFilterVariant=InternalTs  TsampNgainVariant=Passthrough  TsampIntegralVariant=Disabled_SignalSpec  ExternalSaturationOutDataTypeStr=Inherit: Same as second input
  Permanent Magnet Synchronous Machine1 : spsPermanentMagnetSynchronousMachineLib/Permanent Magnet Synchronous Machine  NbPhases=3  FluxDistribution=Trapezoidal  RotorType=Round  MechanicalLoad=Speed w  PresetModel=No  ShowDetailedParameters=on  MeasurementBus=off  Resistance=0.0485  Inductance=8.5e-3  dqInductances=[8.5e-3,8.5e-3]  La=0.000395  MachineConstant=Flux linkage established by magnets (V.s)  Flux=0.1194  VoltageCst=150.0425  TorqueCst=1.4328  Flat=120  Mechanical=[0.0027 0.0004924 4 0]  PolePairs=6  InitialConditions=[0,0, 0,0]  InitialConditions5ph=[0 0 0 0 0 0]  RefAngle=90 degrees behind phase A axis (modified Park)  IterativeDiscreteModel=Trapezoidal non iterative  TsBlock=-1  TsPowergui=0
  Product : Product
  Saturation1 : Saturate  UpperLimit=10000  LowerLimit=0
  Scope : Scope
  Scope1 : Scope
  Scope2 : Scope  NumInputPorts=2
  Step1 : Step  Time=100  After=200  SampleTime=0
  Sum1 : Sum  Inputs=|+-
  Sum2 : Sum  Inputs=|+-
  Transfer Fcn1 : TransferFcn  Numerator=1  Denominator=[0.8 1]
  gates : Subsystem
  ia : Goto
  Positive : PMIOPort  Side=Left
  Nagative : PMIOPort  Port=2  Side=Left
  Torque : Outport
  wires:
  Bus Selector/3 -> [C]  "<Stator current is_c (A)>"
  Bus Selector2/1 -> Decoder/1(hall)
  [B] -> gates/3(ib)
  gates/1(Gates) -> Inverter/1(Gate_signals)
  Permanent Magnet Synchronous Machine1/1 -> Bus Selector1/1, Bus Selector2/1, Bus Selector/1
  Bus Selector/1 -> ia/1  "<Stator current is_a (A)>"
  Bus Selector/2 -> [B]  "<Stator current is_b (A)>"
  [C] -> gates/4(ic)
  From/1 -> gates/2(ia)
  Bus Selector1/1 -> Transfer Fcn1/1, Scope/1  "<Electromagnetic torque Te (N*m)>"
  Step1/1 -> Permanent Magnet Synchronous Machine1/1
  Decoder/1(ems_abc) -> Product/2
  Product/1 -> gates/1(emf_abc)
  Sum1/1 -> PID Controller/1
  Tref/1 -> Scope2/1, Sum1/1
  Transfer Fcn1/1 -> Saturation1/1
  PID Controller/1 -> Sum2/1
  Sum2/1 -> Product/1
  Saturation1/1 -> Torque/1, Sum1/2, Sum2/2, Scope2/2, Scope1/1
  connections:
  Inverter/LConn1 -- Positive/RConn1
  Inverter/LConn2 -- Nagative/RConn1
  Permanent Magnet Synchronous Machine1/LConn1 -- Inverter/RConn1
  Permanent Magnet Synchronous Machine1/LConn2 -- Inverter/RConn2
  Permanent Magnet Synchronous Machine1/LConn3 -- Inverter/RConn3

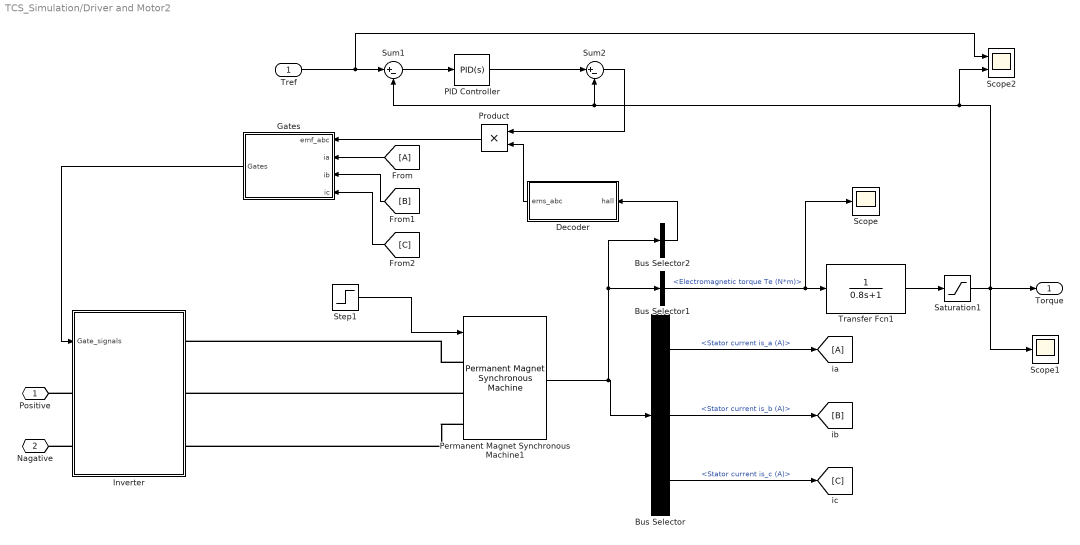
== system TCS_Simulation/Driver and Motor2 ==
  Tref : Inport
  Bus Selector : BusSelector  OutputSignals=Stator current is_a (A),Stator current is_b (A),Stator current is_c (A)
  Bus Selector1 : BusSelector  OutputSignals=Electromagnetic torque Te (N*m)
  Bus Selector2 : BusSelector  OutputSignals=Hall effect signal h_a,Hall effect signal h_b,Hall effect signal h_c  OutputAsBus=on
  Decoder : Subsystem
  From : From
  Gates : Subsystem
  Inverter : Subsystem
  PID Controller : slpidlib/PID Controller  Controller=PID  Form=Parallel  TimeDomain=Continuous-time  UseExternalTs=off  SampleTime=-1  IntegratorMethod=Forward Euler  FilterMethod=Forward Euler  ControllerParametersSource=internal  P=100  I=10  UseKiTs=off  D=1  N=100  UseFilter=on  TunerSelectOption=Transfer Function Based (PID Tuner App)  InitialConditionSource=internal  InitialConditionForIntegrator=0  InitialConditionForFilter=0  DifferentiatorICPrevScaledInput=0  ExternalReset=none  TrackingMode=off  Kt=1  LimitOutput=off  SatLimitsSource=internal  UpperSaturationLimit=inf  LowerSaturationLimit=-inf  LinearizeAsGain=on  AntiWindupMode=none  Kb=1  LimitIntegrator=off  UpperIntegratorSaturationLimit=inf  LowerIntegratorSaturationLimit=-inf  POutMin=[]  POutMax=[]  IOutMin=[]  IOutMax=[]  DOutMin=[]  DOutMax=[]  NOutMin=[]  NOutMax=[]  SumOutMin=[]  SumOutMax=[]  SaturationOutMin=[]  SaturationOutMax=[]  PParamMin=[]  PParamMax=[]  IParamMin=[]  IParamMax=[]  DParamMin=[]  DParamMax=[]  NParamMin=[]  NParamMax=[]  KbParamMin=[]  KbParamMax=[]  KtParamMin=[]  KtParamMax=[]  KbOutMin=[]  KbOutMax=[]  KtOutMin=[]  KtOutMax=[]  IntegratorOutMin=[]  IntegratorOutMax=[]  FilterOutMin=[]  FilterOutMax=[]  SumI1OutMin=[]  SumI1OutMax=[]  SumI2OutMin=[]  SumI2OutMax=[]  SumI3OutMin=[]  SumI3OutMax=[]  SumI4OutMin=[]  SumI4OutMax=[]  SumDOutMin=[]  SumDOutMax=[]  DifferentiatorOutMin=[]  DifferentiatorOutMax=[]  FilterDiffOutCoefMin=[]  FilterDiffOutCoefMax=[]  ReciprocalOutMin=[]  ReciprocalOutMax=[]  SumDenOutMin=[]  SumDenOutMax=[]  SumNumOutMin=[]  SumNumOutMax=[]  DivideOutMin=[]  DivideOutMax=[]  UdiffTsProdOutMin=[]  UdiffTsProdOutMax=[]  NTsProdOutMin=[]  NTsProdOutMax=[]  UintegralTsProdOutMin=[]  UintegralTsProdOutMax=[]  UngainTsProdOutMin=[]  UngainTsProdOutMax=[]  ClampingZeroOutDataTypeStr=Inherit: Inherit via back propagation  ClampingZeroOutMin=[]  ClampingZeroOutMax=[]  FilterDenConstantOutDataTypeStr=Inherit: Inherit via back propagation  FilterDenConstantOutMin=[]  FilterDenConstantOutMax=[]  PCopyOutDataTypeStr=Inherit: Inherit via back propagation  PCopyOutMin=[]  PCopyOutMax=[]  NCopyOutDataTypeStr=Inherit: Inherit via back propagation  NCopyOutMin=[]  NCopyOutMax=[]  IntegratorContinuousStateAttributes=''  IntegratorStateMustResolveToSignalObject=off  IntegratorRTWStateStorageClass=Auto  FilterContinuousStateAttributes=''  FilterStateMustResolveToSignalObject=off  FilterRTWStateStorageClass=Auto  ParallelPVariant=InternalParameters  IdealPVariant=Disabled  IVariant=InternalParameters  DVariant=InternalParameters  IntegratorVariant=Continuous  SatVariant=Disabled  AWVariant=Passthrough  PCopyVariant=Disabled  TRVariant=Disabled  FdbkBlocksVariant=Forward  IdealPFdbkVariant=Disabled  SatFdbkVariant=Disabled  DerivativeFilterVariant=ContFilter  NVariant=InternalParameters  NCopyVariant=Disabled  FilterICVariant=InternalICsFilter  IntegratorICVariant=InternalICs  ExternalResetVariant=Disabled  TRSumVariant=Passthrough  SumFdbkVariant=Disabled  SumVariant=Sum_PID  TsampFilterVariant=InternalTs  TsampNgainVariant=Passthrough  TsampIntegralVariant=Disabled_SignalSpec  ExternalSaturationOutDataTypeStr=Inherit: Same as second input
  Permanent Magnet Synchronous Machine1 : spsPermanentMagnetSynchronousMachineLib/Permanent Magnet Synchronous Machine  NbPhases=3  FluxDistribution=Trapezoidal  RotorType=Round  MechanicalLoad=Speed w  PresetModel=No  ShowDetailedParameters=on  MeasurementBus=off  Resistance=0.0485  Inductance=8.5e-3  dqInductances=[8.5e-3,8.5e-3]  La=0.000395  MachineConstant=Flux linkage established by magnets (V.s)  Flux=0.1194  VoltageCst=150.0425  TorqueCst=1.4328  Flat=120  Mechanical=[0.0027 0.0004924 4 0]  PolePairs=6  InitialConditions=[0,0, 0,0]  InitialConditions5ph=[0 0 0 0 0 0]  RefAngle=90 degrees behind phase A axis (modified Park)  IterativeDiscreteModel=Trapezoidal non iterative  TsBlock=-1  TsPowergui=0
  Product : Product
  Saturation1 : Saturate  UpperLimit=10000  LowerLimit=0
  Scope : Scope
  Scope1 : Scope
  Scope2 : Scope  NumInputPorts=2
  Step1 : Step  Time=100  After=200  SampleTime=0
  Sum1 : Sum  Inputs=|+-
  Sum2 : Sum  Inputs=|+-
  Transfer Fcn1 : TransferFcn  Denominator=[0.8 1]
  ia : Goto
  Positive : PMIOPort  Side=Left
  Nagative : PMIOPort  Port=2  Side=Left
  Torque : Outport
  wires:
  Bus Selector/3 -> [C]  "<Stator current is_c (A)>"
  Bus Selector2/1 -> Decoder/1(hall)
  [B] -> Gates/3(ib)
  Gates/1(Gates) -> Inverter/1(Gate_signals)
  Permanent Magnet Synchronous Machine1/1 -> Bus Selector1/1, Bus Selector2/1, Bus Selector/1
  Bus Selector/1 -> ia/1  "<Stator current is_a (A)>"
  Bus Selector/2 -> [B]  "<Stator current is_b (A)>"
  [C] -> Gates/4(ic)
  From/1 -> Gates/2(ia)
  Bus Selector1/1 -> Transfer Fcn1/1, Scope/1  "<Electromagnetic torque Te (N*m)>"
  Step1/1 -> Permanent Magnet Synchronous Machine1/1
  Decoder/1(ems_abc) -> Product/2
  Product/1 -> Gates/1(emf_abc)
  Sum1/1 -> PID Controller/1
  Tref/1 -> Scope2/1, Sum1/1
  PID Controller/1 -> Sum2/1
  Sum2/1 -> Product/1
  Transfer Fcn1/1 -> Saturation1/1
  Saturation1/1 -> Torque/1, Sum1/2, Sum2/2, Scope2/2, Scope1/1
  connections:
  Inverter/LConn1 -- Positive/RConn1
  Inverter/LConn2 -- Nagative/RConn1
  Permanent Magnet Synchronous Machine1/LConn1 -- Inverter/RConn1
  Permanent Magnet Synchronous Machine1/LConn2 -- Inverter/RConn2
  Permanent Magnet Synchronous Machine1/LConn3 -- Inverter/RConn3

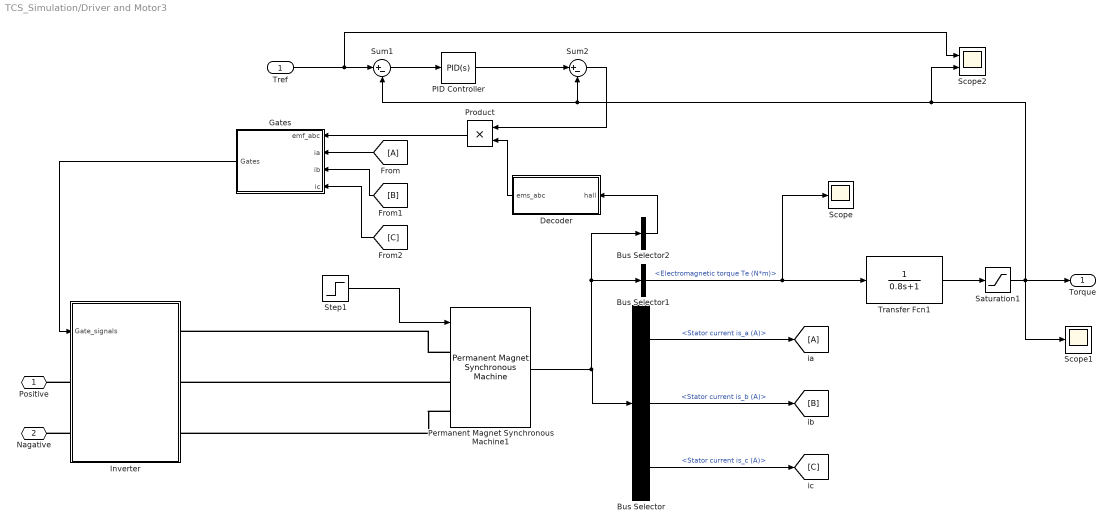
== system TCS_Simulation/Driver and Motor3 ==
  Tref : Inport
  Bus Selector : BusSelector  OutputSignals=Stator current is_a (A),Stator current is_b (A),Stator current is_c (A)
  Bus Selector1 : BusSelector  OutputSignals=Electromagnetic torque Te (N*m)
  Bus Selector2 : BusSelector  OutputSignals=Hall effect signal h_a,Hall effect signal h_b,Hall effect signal h_c  OutputAsBus=on
  Decoder : Subsystem
  From : From
  Gates : Subsystem
  Inverter : Subsystem
  PID Controller : slpidlib/PID Controller  Controller=PID  Form=Parallel  TimeDomain=Continuous-time  UseExternalTs=off  SampleTime=-1  IntegratorMethod=Forward Euler  FilterMethod=Forward Euler  ControllerParametersSource=internal  P=100  I=10  UseKiTs=off  D=1  N=100  UseFilter=on  TunerSelectOption=Transfer Function Based (PID Tuner App)  InitialConditionSource=internal  InitialConditionForIntegrator=0  InitialConditionForFilter=0  DifferentiatorICPrevScaledInput=0  ExternalReset=none  TrackingMode=off  Kt=1  LimitOutput=off  SatLimitsSource=internal  UpperSaturationLimit=inf  LowerSaturationLimit=-inf  LinearizeAsGain=on  AntiWindupMode=none  Kb=1  LimitIntegrator=off  UpperIntegratorSaturationLimit=inf  LowerIntegratorSaturationLimit=-inf  POutMin=[]  POutMax=[]  IOutMin=[]  IOutMax=[]  DOutMin=[]  DOutMax=[]  NOutMin=[]  NOutMax=[]  SumOutMin=[]  SumOutMax=[]  SaturationOutMin=[]  SaturationOutMax=[]  PParamMin=[]  PParamMax=[]  IParamMin=[]  IParamMax=[]  DParamMin=[]  DParamMax=[]  NParamMin=[]  NParamMax=[]  KbParamMin=[]  KbParamMax=[]  KtParamMin=[]  KtParamMax=[]  KbOutMin=[]  KbOutMax=[]  KtOutMin=[]  KtOutMax=[]  IntegratorOutMin=[]  IntegratorOutMax=[]  FilterOutMin=[]  FilterOutMax=[]  SumI1OutMin=[]  SumI1OutMax=[]  SumI2OutMin=[]  SumI2OutMax=[]  SumI3OutMin=[]  SumI3OutMax=[]  SumI4OutMin=[]  SumI4OutMax=[]  SumDOutMin=[]  SumDOutMax=[]  DifferentiatorOutMin=[]  DifferentiatorOutMax=[]  FilterDiffOutCoefMin=[]  FilterDiffOutCoefMax=[]  ReciprocalOutMin=[]  ReciprocalOutMax=[]  SumDenOutMin=[]  SumDenOutMax=[]  SumNumOutMin=[]  SumNumOutMax=[]  DivideOutMin=[]  DivideOutMax=[]  UdiffTsProdOutMin=[]  UdiffTsProdOutMax=[]  NTsProdOutMin=[]  NTsProdOutMax=[]  UintegralTsProdOutMin=[]  UintegralTsProdOutMax=[]  UngainTsProdOutMin=[]  UngainTsProdOutMax=[]  ClampingZeroOutDataTypeStr=Inherit: Inherit via back propagation  ClampingZeroOutMin=[]  ClampingZeroOutMax=[]  FilterDenConstantOutDataTypeStr=Inherit: Inherit via back propagation  FilterDenConstantOutMin=[]  FilterDenConstantOutMax=[]  PCopyOutDataTypeStr=Inherit: Inherit via back propagation  PCopyOutMin=[]  PCopyOutMax=[]  NCopyOutDataTypeStr=Inherit: Inherit via back propagation  NCopyOutMin=[]  NCopyOutMax=[]  IntegratorContinuousStateAttributes=''  IntegratorStateMustResolveToSignalObject=off  IntegratorRTWStateStorageClass=Auto  FilterContinuousStateAttributes=''  FilterStateMustResolveToSignalObject=off  FilterRTWStateStorageClass=Auto  ParallelPVariant=InternalParameters  IdealPVariant=Disabled  IVariant=InternalParameters  DVariant=InternalParameters  IntegratorVariant=Continuous  SatVariant=Disabled  AWVariant=Passthrough  PCopyVariant=Disabled  TRVariant=Disabled  FdbkBlocksVariant=Forward  IdealPFdbkVariant=Disabled  SatFdbkVariant=Disabled  DerivativeFilterVariant=ContFilter  NVariant=InternalParameters  NCopyVariant=Disabled  FilterICVariant=InternalICsFilter  IntegratorICVariant=InternalICs  ExternalResetVariant=Disabled  TRSumVariant=Passthrough  SumFdbkVariant=Disabled  SumVariant=Sum_PID  TsampFilterVariant=InternalTs  TsampNgainVariant=Passthrough  TsampIntegralVariant=Disabled_SignalSpec  ExternalSaturationOutDataTypeStr=Inherit: Same as second input
  Permanent Magnet Synchronous Machine1 : spsPermanentMagnetSynchronousMachineLib/Permanent Magnet Synchronous Machine  NbPhases=3  FluxDistribution=Trapezoidal  RotorType=Round  MechanicalLoad=Speed w  PresetModel=No  ShowDetailedParameters=on  MeasurementBus=off  Resistance=0.0485  Inductance=8.5e-3  dqInductances=[8.5e-3,8.5e-3]  La=0.000395  MachineConstant=Flux linkage established by magnets (V.s)  Flux=0.1194  VoltageCst=150.0425  TorqueCst=1.4328  Flat=120  Mechanical=[0.0027 0.0004924 4 0]  PolePairs=6  InitialConditions=[0,0, 0,0]  InitialConditions5ph=[0 0 0 0 0 0]  RefAngle=90 degrees behind phase A axis (modified Park)  IterativeDiscreteModel=Trapezoidal non iterative  TsBlock=-1  TsPowergui=0
  Product : Product
  Saturation1 : Saturate  UpperLimit=10000  LowerLimit=0
  Scope : Scope
  Scope1 : Scope
  Scope2 : Scope  NumInputPorts=2
  Step1 : Step  Time=100  After=200  SampleTime=0
  Sum1 : Sum  Inputs=|+-
  Sum2 : Sum  Inputs=|+-
  Transfer Fcn1 : TransferFcn  Denominator=[0.8 1]
  ia : Goto
  Positive : PMIOPort  Side=Left
  Nagative : PMIOPort  Port=2  Side=Left
  Torque : Outport
  wires:
  Bus Selector/3 -> [C]  "<Stator current is_c (A)>"
  Bus Selector2/1 -> Decoder/1(hall)
  [B] -> Gates/3(ib)
  Gates/1(Gates) -> Inverter/1(Gate_signals)
  Permanent Magnet Synchronous Machine1/1 -> Bus Selector1/1, Bus Selector2/1, Bus Selector/1
  Bus Selector/1 -> ia/1  "<Stator current is_a (A)>"
  Bus Selector/2 -> [B]  "<Stator current is_b (A)>"
  [C] -> Gates/4(ic)
  From/1 -> Gates/2(ia)
  Bus Selector1/1 -> Transfer Fcn1/1, Scope/1  "<Electromagnetic torque Te (N*m)>"
  Step1/1 -> Permanent Magnet Synchronous Machine1/1
  Decoder/1(ems_abc) -> Product/2
  Product/1 -> Gates/1(emf_abc)
  Sum1/1 -> PID Controller/1
  Tref/1 -> Scope2/1, Sum1/1
  PID Controller/1 -> Sum2/1
  Sum2/1 -> Product/1
  Transfer Fcn1/1 -> Saturation1/1
  Saturation1/1 -> Torque/1, Sum1/2, Sum2/2, Scope2/2, Scope1/1
  connections:
  Inverter/LConn1 -- Positive/RConn1
  Inverter/LConn2 -- Nagative/RConn1
  Permanent Magnet Synchronous Machine1/LConn1 -- Inverter/RConn1
  Permanent Magnet Synchronous Machine1/LConn2 -- Inverter/RConn2
  Permanent Magnet Synchronous Machine1/LConn3 -- Inverter/RConn3

== system TCS_Simulation/High Torque ==
  Demux : Demux  Tag=STV Demux  Outputs=1
      settings: DisplayOption=none
  FromWs : FromWorkspace  Tag=STV FromWs  VariableName=tuvar
      SigBuilderData=|
      | common.afterFinalStr = 'Extrapolate'
      | common.sampleTime = 0
      | dataSet.timeRange = [0 10]
      | dataSet.name = 'Group 1'
      | sbobj.Groups.Name = 'Group 1'
      | sbobj.Groups.Signals.Name = 'Signal 1'
      | sbobj.Groups.Signals.XData = [0 0.5 1.5 2.2 4 10]
      | sbobj.Groups.Signals.YData = [0 40 120 120 120 120]
  Signal 1 : Outport  Tag=STV Outport
  wires:
  FromWs/1 -> Demux/1
  Demux/1 -> Signal 1/1

== system TCS_Simulation/PID control ==
  lamda : Inport
  Constant : Constant  Value=0
  Constant1 : Constant
  PID Controller : slpidlib/PID Controller  Controller=PID  Form=Parallel  TimeDomain=Discrete-time  UseExternalTs=off  SampleTime=-1  IntegratorMethod=Forward Euler  FilterMethod=Forward Euler  ControllerParametersSource=internal  P=30  I=0.5  UseKiTs=off  D=20  N=100  UseFilter=off  TunerSelectOption=Transfer Function Based (PID Tuner App)  InitialConditionSource=internal  InitialConditionForIntegrator=0  InitialConditionForFilter=0  DifferentiatorICPrevScaledInput=0  ExternalReset=none  TrackingMode=off  Kt=1  LimitOutput=on  SatLimitsSource=internal  UpperSaturationLimit=1  LowerSaturationLimit=0  LinearizeAsGain=off  AntiWindupMode=none  Kb=1  LimitIntegrator=off  UpperIntegratorSaturationLimit=1  LowerIntegratorSaturationLimit=0  POutMin=[]  POutMax=[]  IOutMin=[]  IOutMax=[]  DOutMin=[]  DOutMax=[]  NOutMin=[]  NOutMax=[]  SumOutMin=[]  SumOutMax=[]  SaturationOutMin=[]  SaturationOutMax=[]  PParamMin=[]  PParamMax=[]  IParamMin=[]  IParamMax=[]  DParamMin=[]  DParamMax=[]  NParamMin=[]  NParamMax=[]  KbParamMin=[]  KbParamMax=[]  KtParamMin=[]  KtParamMax=[]  KbOutMin=[]  KbOutMax=[]  KtOutMin=[]  KtOutMax=[]  IntegratorOutMin=[]  IntegratorOutMax=[]  FilterOutMin=[]  FilterOutMax=[]  SumI1OutMin=[]  SumI1OutMax=[]  SumI2OutMin=[]  SumI2OutMax=[]  SumI3OutMin=[]  SumI3OutMax=[]  SumI4OutMin=[]  SumI4OutMax=[]  SumDOutMin=[]  SumDOutMax=[]  DifferentiatorOutMin=[]  DifferentiatorOutMax=[]  FilterDiffOutCoefMin=[]  FilterDiffOutCoefMax=[]  ReciprocalOutMin=[]  ReciprocalOutMax=[]  SumDenOutMin=[]  SumDenOutMax=[]  SumNumOutMin=[]  SumNumOutMax=[]  DivideOutMin=[]  DivideOutMax=[]  UdiffTsProdOutMin=[]  UdiffTsProdOutMax=[]  NTsProdOutMin=[]  NTsProdOutMax=[]  UintegralTsProdOutMin=[]  UintegralTsProdOutMax=[]  UngainTsProdOutMin=[]  UngainTsProdOutMax=[]  ClampingZeroOutDataTypeStr=Inherit: Inherit via back propagation  ClampingZeroOutMin=[]  ClampingZeroOutMax=[]  FilterDenConstantOutDataTypeStr=Inherit: Inherit via back propagation  FilterDenConstantOutMin=[]  FilterDenConstantOutMax=[]  PCopyOutDataTypeStr=Inherit: Inherit via back propagation  PCopyOutMin=[]  PCopyOutMax=[]  NCopyOutDataTypeStr=Inherit: Inherit via back propagation  NCopyOutMin=[]  NCopyOutMax=[]  IntegratorContinuousStateAttributes=''  IntegratorStateMustResolveToSignalObject=off  IntegratorRTWStateStorageClass=Auto  FilterContinuousStateAttributes=''  FilterStateMustResolveToSignalObject=off  FilterRTWStateStorageClass=Auto  ParallelPVariant=InternalParameters  IdealPVariant=Disabled  IVariant=InternalParameters  DVariant=InternalParameters  IntegratorVariant=Discrete  SatVariant=Enabled  AWVariant=Passthrough  PCopyVariant=Disabled  TRVariant=Disabled  FdbkBlocksVariant=Forward  IdealPFdbkVariant=Disabled  SatFdbkVariant=Disabled  DerivativeFilterVariant=Differentiator  NVariant=Passthrough  NCopyVariant=Disabled_SignalSpec  FilterICVariant=InternalICsDifferentiator  IntegratorICVariant=InternalICs  ExternalResetVariant=Disabled  TRSumVariant=Passthrough  SumFdbkVariant=Disabled  SumVariant=Sum_PID  TsampFilterVariant=InternalTs  TsampNgainVariant=Passthrough  TsampIntegralVariant=Disabled_SignalSpec  ExternalSaturationOutDataTypeStr=Inherit: Same as second input
  Sum2 : Sum  Inputs=|+-
  Switch1 : Switch  Threshold=0.2  SaturateOnIntegerOverflow=off  InputSameDT=off
  s : Outport
  wires:
  Constant1/1 -> Switch1/3
  Constant/1 -> Sum2/1
  lamda/1 -> Switch1/2, Sum2/2
  Sum2/1 -> PID Controller/1
  Switch1/1 -> s/1
  PID Controller/1 -> Switch1/1
